simulink model "PendulumProjectMU"  (R2022b)
settings: Solver=FixedStepAuto  StartTime=0.0  StopTime=inf  FixedStep=0.01  RelTol=1e-3
model workspace (MATLAB code in the model file):
  | %Parameters from hardware:
  | Mc = 0.540 + 0.048;% [kg]mass of cart
  | l = 0.49; % [m] Pendelum length
  | Lcg = l/2; % [m] lenght to center of mass
  | m = 0.022;% [kg] Mass of pendelum rod
  | g = 9.81; % m/s^2
  | 
  | %Motor parameters (some estimates, some from Sonali):
  | Rm = 1.3;%[ohm] motor armature resistence
  | kb = 0.02;%[vs/rad]back emf constant
  | kt = 0.02;%[vs/rad]motor touque constant
  | r =  0.04/(2*pi); %[m]radius pulley motor (and encoder)
  | 
  | %Very rough estimate:
  | c = 5; %[N/(m/s)] viscous friction cart
  | b = 0.00001;% [Nm/rad/s]Viscous damping pendelum
  | I = 0.00007; % [kgm^2]
  | 
  | %FOR CASE LOGIC SIMULINK MODEL:
  | offset= 15;% degrees Ofsett from pi, before pendelum control takes over for swing up
  | highThetaTreshold = pi+ pi*offset/180;
  | lowThetaTreshold = pi- pi*offset/180;
  | 
  | %Theshold values to stop cart if close to edges
  | xMAX = 0.25;
  | xMIN = -0.25;
libraries: arduinolib x8, simulink x2, arduinosensorlib x2
settings Model: FPTRunName=Active  ExtModeTrigDuration=2  Creator=The MathWorks, Inc.  LastModifiedBy=Bruker
settings SolverCC: AlgebraicLoopSolver=TrustRegion
settings DataIOCC: LimitDataPoints=on  ReturnWorkspaceOutputs=off
settings OptimizationCC: ExpressionDepthLimit=2147483647  LifeSpan=Inf  MaxStackSize=64
settings DebuggingCC: UnderspecifiedInitializationDetection=Classic  MergeDetectMultiDrivingBlocksExec=none  FcnCallInpInsideContextMsg=warning  UnconnectedInputMsg=warning  UnconnectedOutputMsg=warning  UnconnectedLineMsg=warning  AllowSymbolicDim=off  StateNameClashWarn=warning  SFUnexpectedBacktrackingDiag=warning  SFNoUnconditionalDefaultTransitionDiag=warning  SFExecutionAtInitializationDiag=none  SFMachineParentedDataDiag=warning  ArithmeticOperatorsInVariantConditions=warning
settings HardwareCC: ProdBitPerInt=16  ProdBitPerPointer=16  ProdBitPerSizeT=16  ProdBitPerPtrDiffT=16  ProdLargestAtomicFloat=None  ProdWordSize=8  ProdHWDeviceType=Atmel->AVR  UseEmbeddedCoderFeatures=off  UseSimulinkCoderFeatures=off
settings ModelReferenceCC: EnableRefExpFcnMdlSchedulingChecks=on
settings SFSimCC: SimUseLocalCustomCode=off  MATLABDynamicMemAlloc=off
settings RTWCC: Description=Embedded Coder  SystemTargetFile=ert.tlc  HardwareBoard=Arduino Mega 2560  TemplateMakefile=ert_default_tmf  GenerateReport=on  RTWVerbose=off  RTWUseLocalCustomCode=off  Toolchain=Arduino AVR  BuildConfiguration=Faster Runs  LaunchReport=on  DLArmComputeVersion=19.05
settings CodeAppCC: ForceParamTrailComments=on  OperatorAnnotations=on  MangleLength=10  StateflowObjectComments=on  MATLABSourceComments=on
settings ERTTargetCC: MultiwordLength=2048  ERTCustomFileBanners=off  SupportContinuousTime=on  SupportNonInlinedSFcns=on  RemoveResetFunc=off  ModelStepFunctionPrototypeControlCompliant=off
settings ConfigComp: CovMetricSettings=dw  CovSaveCumulativeToWorkspaceVar=on  CovSaveSingleToWorkspaceVar=on  CovExternalEMLEnable=off  CovSFcnEnable=off

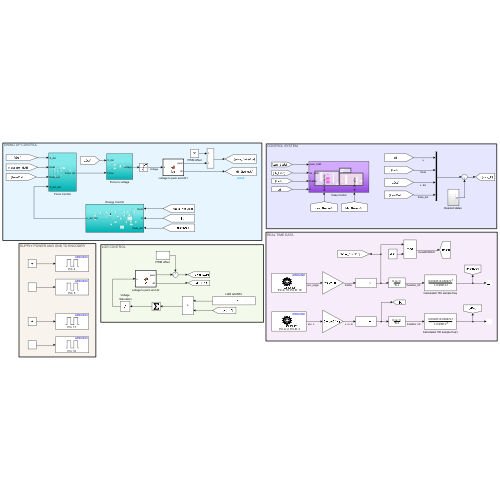
[thumbnail: Simulink's stored preview of the top-level diagram]
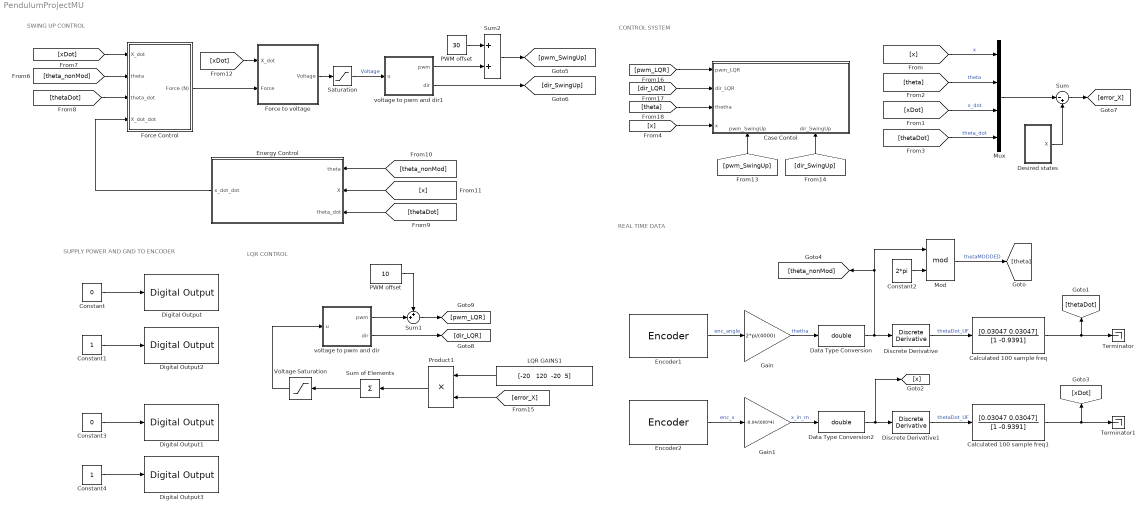
== system PendulumProjectMU ==
  note: LQR CONTROL
  note: SWING UP CONTROL
  note: CONTROL SYSTEM
  note: REAL TIME DATA
  note: SUPPLY POWER AND GND TO ENCODER
  Calculated 100 sample freq : DiscreteFilter  Numerator=[0.03047 0.03047]  Denominator=[1 -0.9391]  SampleTime=0.01
  Calculated 100 sample freq1 : DiscreteFilter  Numerator=[0.03047 0.03047]  Denominator=[1 -0.9391]  SampleTime=0.01
  Case Contol : Subsystem
      settings: PortSchema="{\"entries\":[{\"content\":{\"sides\":[{\"content\":{\"connectorIds\":[\"In1\",\"In2\",\"In3\",\"In4\"]},\"type\":\"ConnectorPlacement.EquallySpacedRectSide\",\"uuid\":\"b9c187f4-b904-4d2f-9cde-60dd328b1521\"},{\"content\":{\"connectorIds\":[],\"side\":\"RIGHT\"},\"type\":\"ConnectorPlacement.EquallySpacedRectSide\",\"uuid\":\"bc2320ec-c90b-418d-8662-363a4a51a6b8\"},{\"content\":{\"connectorIds\":[],\"side\":\"TOP\"},\"type\":\"ConnectorPlacement.EquallySpacedRectSide\",\"uuid\":\"d413f3a0-4126-4ff6-b863-89d2afe3c2f6\"},{\"content\":{\"connectorIds\":[\"In5\",\"In6\"],\"side\":\"BOTTOM\"},\"type\":\"ConnectorPlacement.EquallySpacedRectSide\",\"uuid\":\"5bcc0f4c-eb85-4f39-a4e6-dc5e871715b7\"}]},\"type\":\"ConnectorPlacement.EquallySpacedConnector\",\"uuid\":\"881b5d2a-3ec5-43c5-91bc-30ecaf4ea49e\"}],\"packageUris\":[\"http://schema.mathworks.com/mf0/Connector/R2020b\"],\"version\":\"1.0\"}"
  Constant : Constant  Value=0
  Constant1 : Constant
  Constant2 : Constant  Value=2*pi
  Constant3 : Constant  Value=0
  Constant4 : Constant
  Data Type Conversion : DataTypeConversion  OutDataTypeStr=double  SaturateOnIntegerOverflow=off  RndMeth=Floor
  Data Type Conversion2 : DataTypeConversion  OutDataTypeStr=double  SaturateOnIntegerOverflow=off  RndMeth=Floor
  "Desired states " : Subsystem
  Digital Output : arduinolib/Digital Output  pinNumber=4  Direction=output  blockPlatform=arduino
  Digital Output1 : arduinolib/Digital Output  pinNumber=17  Direction=output  blockPlatform=arduino
  Digital Output2 : arduinolib/Digital Output  pinNumber=5  Direction=output  blockPlatform=arduino
  Digital Output3 : arduinolib/Digital Output  pinNumber=16  Direction=output  blockPlatform=arduino
  Discrete Derivative : simulink/Quick Insert/Discrete/Discrete Derivative  gainval=1.0  ICPrevScaledInput=0.0  OutMin=[]  OutMax=[]  OutDataType=fixdt(1, 16)  OutScaling=2^-10  DoSatur=off
  Discrete Derivative1 : simulink/Quick Insert/Discrete/Discrete Derivative  gainval=1.0  ICPrevScaledInput=0.0  OutMin=[]  OutMax=[]  OutDataType=fixdt(1, 16)  OutScaling=2^-10  DoSatur=off
  Encoder1 : arduinosensorlib/Encoder  InputA=19  InputB=18  Mode=No reset  SampleTime=0.01
  Encoder2 : arduinosensorlib/Encoder  InputA=2  InputB=3  Mode=No reset  SampleTime=0.01
  Energy Control : Subsystem
  Force Control : Subsystem
  Force to voltage : Subsystem
  Gain : Gain  Gain=2*pi/(4000)
  Gain1 : Gain  Gain=-0.04/(600*4)
  LQR GAINS1 : Constant  Value="[-20   120  -20  5]"
  Mod : Math  Operator=mod  SignedPower=on
  Mux : Mux
  PWM offset : Constant  Value=30
  "PWM offset " : Constant  Value=10
  Product1 : Product
  Saturation : Saturate  UpperLimit=3.2  LowerLimit=-3.2
  Sum : Sum  Inputs=|-+
  Sum of Elements : Sum  Inputs=+
  Sum1 : Sum  Inputs=++|
  Sum2 : Sum
  Terminator : Terminator
  Terminator1 : Terminator
  Voltage Saturation : Saturate  UpperLimit=6  LowerLimit=-6
  voltage to pwm and dir : MATLAB Function  TreatAsAtomicUnit=on
  voltage to pwm and dir1 : MATLAB Function  TreatAsAtomicUnit=on
  wires:
  Encoder1/1 -> Gain/1  "enc_angle"
  Constant/1 -> Digital Output/1
  Constant1/1 -> Digital Output2/1
  Gain/1 -> Data Type Conversion/1  "thetha"
  Encoder2/1 -> Gain1/1  "enc_x"
  Constant3/1 -> Digital Output1/1
  Constant4/1 -> Digital Output3/1
  Gain1/1 -> Data Type Conversion2/1  "x_in_m"
  [theta] -> Mux/2  "theta"
  [x] -> Mux/1  "x"
  Mux/1 -> Sum/1
  [xDot] -> Mux/3  "x_dot"
  [thetaDot] -> Mux/4  "theta_dot"
  Data Type Conversion2/1 -> Discrete Derivative1/1, [x]
  Voltage Saturation/1 -> voltage to pwm and dir/1(u)
  voltage to pwm and dir/1(pwm) -> Sum1/2
  "PWM offset "/1 -> Sum1/1
  Calculated 100 sample freq1/1 -> [xDot], Terminator1/1
  Calculated 100 sample freq/1 -> [thetaDot], Terminator/1
  Discrete Derivative/1 -> Calculated 100 sample freq/1  "thetaDot_UF"
  Discrete Derivative1/1 -> Calculated 100 sample freq1/1  "thetaDot_UF"
  "Desired states "/1(X) -> Sum/2
  [theta] -> Case Contol/3(thetha)
  Data Type Conversion/1 -> Discrete Derivative/1, Mod/1, [theta_nonMod]
  Mod/1 -> [theta]  "thetaMODDED"
  [x] -> Case Contol/4(x)
  Force to voltage/1(Voltage) -> Saturation/1
  Energy Control/1(x_dot_dot) -> Force Control/4(X_dot_dot)
  Force Control/1(Force (N)) -> Force to voltage/2(Force)
  [theta_nonMod] -> Force Control/2(theta)
  [xDot] -> Force Control/1(X_dot)
  [thetaDot] -> Force Control/3(theta_dot)
  [thetaDot] -> Energy Control/3(theta_dot)
  [theta_nonMod] -> Energy Control/1(theta)
  [x] -> Energy Control/2(X)
  [xDot] -> Force to voltage/1(X_dot)
  Saturation/1 -> voltage to pwm and dir1/1(u)  "Voltage"
  Product1/1 -> Sum of Elements/1
  LQR GAINS1/1 -> Product1/1
  Sum of Elements/1 -> Voltage Saturation/1
  PWM offset/1 -> Sum2/1
  voltage to pwm and dir1/1(pwm) -> Sum2/2
  Sum2/1 -> [pwm_SwingUp]
  voltage to pwm and dir1/2(dir) -> [dir_SwingUp]
  [pwm_SwingUp] -> Case Contol/5(pwm_SwingUp)
  [dir_SwingUp] -> Case Contol/6(dir_SwingUp)
  Sum/1 -> [error_X]
  [error_X] -> Product1/2
  voltage to pwm and dir/2(dir) -> [dir_LQR]
  Sum1/1 -> [pwm_LQR]
  [pwm_LQR] -> Case Contol/1(pwm_LQR)
  [dir_LQR] -> Case Contol/2("dir_LQR ")
  Constant2/1 -> Mod/2

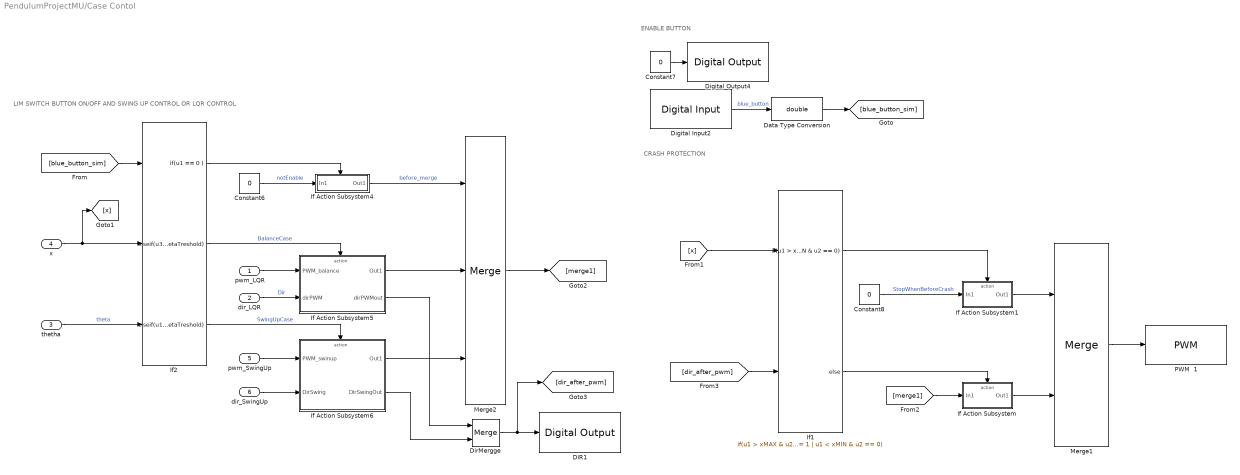
== system PendulumProjectMU/Case Contol ==
  note: CRASH PROTECTION
  note: ENABLE BUTTON
  note: LIM SWITCH BUTTON ON/OFF AND SWING UP CONTROL OR LQR CONTROL
  pwm_LQR : Inport
  "dir_LQR " : Inport  Port=2
  thetha : Inport  Port=3
  x : Inport  Port=4
  pwm_SwingUp : Inport  Port=5
  dir_SwingUp : Inport  Port=6
  Constant6 : Constant  Value=0
  Constant7 : Constant  Value=0
  Constant8 : Constant  Value=0
  DIR1 : arduinolib/Digital Output  pinNumber=12  Direction=output  blockPlatform=arduino
  Data Type Conversion : DataTypeConversion  OutDataTypeStr=double  SaturateOnIntegerOverflow=off  RndMeth=Floor
  Digital Input2 : arduinolib/Digital Input  pinNumber=42  mode=Input Pullup  Direction=input  SampleTime=0.01  blockPlatform=arduino
  Digital Output4 : arduinolib/Digital Output  pinNumber=43  Direction=output  blockPlatform=arduino
  DirMergge : Merge
  If Action Subsystem : Subsystem  TreatAsAtomicUnit=on
  If Action Subsystem1 : Subsystem  TreatAsAtomicUnit=on
  If Action Subsystem4 : Subsystem  TreatAsAtomicUnit=on
  If Action Subsystem5 : Subsystem  TreatAsAtomicUnit=on
  If Action Subsystem6 : Subsystem  TreatAsAtomicUnit=on
  If1 : If  NumInputs=2  IfExpression=u1 > xMAX & u2 == 1 | u1 < xMIN & u2 == 0
  If2 : If  NumInputs=3  IfExpression=u1 == 0  ElseIfExpressions="u3 < highThetaTreshold & u3 > lowThetaTreshold  , u1 ~= 0  & u3 > highThetaTreshold | u3 < lowThetaTreshold"  ShowElse=off
  Merge1 : Merge
  Merge2 : Merge  Inputs=3
  PWM  1 : arduinolib/PWM  pinNumber=13  frequencyType=Default  desiredFrequency=490.2  achievableFrequency=490.2
  wires:
  Constant7/1 -> Digital Output4/1
  If2/3 -> If Action Subsystem6/Action  "SwingUpCase"
  If Action Subsystem4/1(Out1) -> Merge2/1  "before_merge"
  If2/1 -> If Action Subsystem4/Action
  Constant6/1 -> If Action Subsystem4/1(In1)  "notEnable"
  Digital Input2/1 -> Data Type Conversion/1  "blue_button"
  If Action Subsystem6/1(Out1) -> Merge2/3
  If Action Subsystem5/1(Out1) -> Merge2/2
  thetha/1 -> If2/3  "theta"
  pwm_LQR/1 -> If Action Subsystem5/1(PWM_balance)
  x/1 -> [x], If2/2
  pwm_SwingUp/1 -> If Action Subsystem6/1(PWM_swinup)
  "dir_LQR "/1 -> If Action Subsystem5/2(dirPWM)  "Dir"
  dir_SwingUp/1 -> If Action Subsystem6/2(DirSwing)
  If Action Subsystem5/2(dirPWMout) -> DirMergge/1
  If Action Subsystem6/2(DirSwingOut) -> DirMergge/2
  If1/1 -> If Action Subsystem1/Action
  Constant8/1 -> If Action Subsystem1/1(In1)  "StopWhenBeforeCrash"
  If1/2 -> If Action Subsystem/Action
  If Action Subsystem1/1(Out1) -> Merge1/1
  If Action Subsystem/1(Out1) -> Merge1/2
  Merge1/1 -> PWM  1/1
  If2/2 -> If Action Subsystem5/Action  "BalanceCase"
  Data Type Conversion/1 -> [blue_button_sim]
  [blue_button_sim] -> If2/1
  [x] -> If1/1
  Merge2/1 -> [merge1]
  [merge1] -> If Action Subsystem/1(In1)
  [dir_after_pwm] -> If1/2
  DirMergge/1 -> [dir_after_pwm], DIR1/1

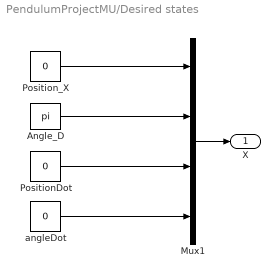
== system PendulumProjectMU/Desired states  ==
  Angle_D : Constant  Value=pi
  Mux1 : Mux
  PositionDot : Constant  Value=0
  Position_X : Constant  Value=0
  angleDot : Constant  Value=0
  X : Outport  VectorParamsAs1DForOutWhenUnconnected=off
  wires:
  Position_X/1 -> Mux1/1
  Angle_D/1 -> Mux1/2
  angleDot/1 -> Mux1/4
  PositionDot/1 -> Mux1/3
  Mux1/1 -> X/1

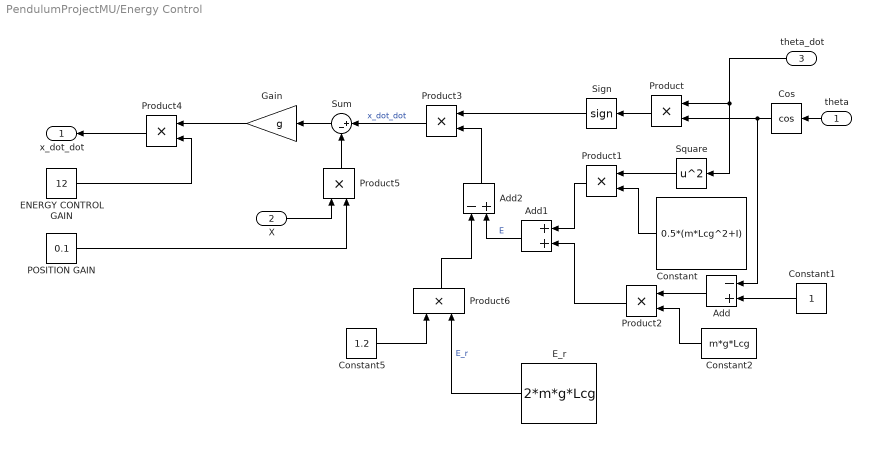
== system PendulumProjectMU/Energy Control ==
  theta : Inport
  X : Inport  Port=2
  theta_dot : Inport  Port=3
  Add : Sum  Inputs=-+
  Add1 : Sum
  Add2 : Sum  Inputs=-+
  Constant : Constant  Value=0.5*(m*Lcg^2+I)  SampleTime=0.01
  Constant1 : Constant  SampleTime=0.01
  Constant2 : Constant  Value=m*g*Lcg
  Constant5 : Constant  Value=1.2  SampleTime=0.01
  Cos : Trigonometry  Operator=cos
  ENERGY CONTROL GAIN : Constant  Value=12  SampleTime=0.01
  E_r : Constant  Value=2*m*g*Lcg  SampleTime=0.01
  Gain : Gain  Gain=g
  POSITION GAIN : Constant  Value=0.1  SampleTime=0.01
  Product{,1..6} (7 alike) : Product
  Sign : Signum
  Square : Math  Operator=square
  Sum : Sum  Inputs=|+-
  x_dot_dot : Outport
  wires:
  E_r/1 -> Product6/2  "E_r"
  Constant/1 -> Product1/2
  Sign/1 -> Product3/1
  Constant2/1 -> Product2/2
  theta_dot/1 -> Square/1, Product/1
  Add/1 -> Product2/1
  Product/1 -> Sign/1
  Add1/1 -> Add2/2  "E"
  Cos/1 -> Product/2, Add/1
  Square/1 -> Product1/1
  Constant1/1 -> Add/2
  Product2/1 -> Add1/2
  Product1/1 -> Add1/1
  Add2/1 -> Product3/2
  theta/1 -> Cos/1
  Product4/1 -> x_dot_dot/1
  Sum/1 -> Gain/1
  Product3/1 -> Sum/1  "x_dot_dot"
  X/1 -> Product5/1
  Product6/1 -> Add2/1
  Product5/1 -> Sum/2
  POSITION GAIN/1 -> Product5/2
  Constant5/1 -> Product6/1
  Gain/1 -> Product4/1
  ENERGY CONTROL GAIN/1 -> Product4/2

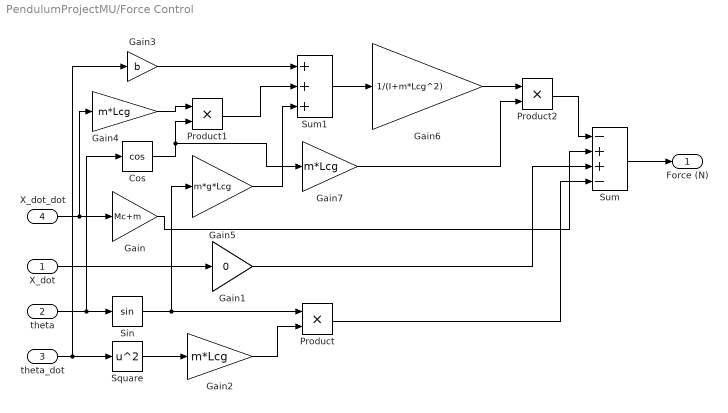
== system PendulumProjectMU/Force Control ==
  X_dot : Inport
  theta : Inport  Port=2
  theta_dot : Inport  Port=3
  X_dot_dot : Inport  Port=4
  Cos : Trigonometry  Operator=cos
  Gain : Gain  Gain=Mc+m
  Gain1 : Gain  Gain=0
  Gain2 : Gain  Gain=m*Lcg
  Gain3 : Gain  Gain=b
  Gain4 : Gain  Gain=m*Lcg
  Gain5 : Gain  Gain=m*g*Lcg
  Gain6 : Gain  Gain=1/(I+m*Lcg^2)
  Gain7 : Gain  Gain=m*Lcg
  Product : Product
  Product1 : Product
  Product2 : Product
  Sin : Trigonometry
  Square : Math  Operator=square
  Sum : Sum  Inputs=-++-
  Sum1 : Sum  Inputs=+++
  Force (N) : Outport  VectorParamsAs1DForOutWhenUnconnected=off
  wires:
  X_dot_dot/1 -> Gain/1, Gain4/1
  X_dot/1 -> Gain1/1
  Square/1 -> Gain2/1
  theta/1 -> Cos/1, Sin/1
  Sin/1 -> Gain5/1, Product/1
  Gain2/1 -> Product/2
  Product/1 -> Sum/4
  Gain1/1 -> Sum/3
  Gain/1 -> Sum/2
  Gain3/1 -> Sum1/1
  Gain4/1 -> Product1/1
  Cos/1 -> Gain7/1, Product1/2
  theta_dot/1 -> Square/1, Gain3/1
  Product1/1 -> Sum1/2
  Gain5/1 -> Sum1/3
  Sum1/1 -> Gain6/1
  Gain6/1 -> Product2/1
  Gain7/1 -> Product2/2
  Product2/1 -> Sum/1
  Sum/1 -> Force (N)/1

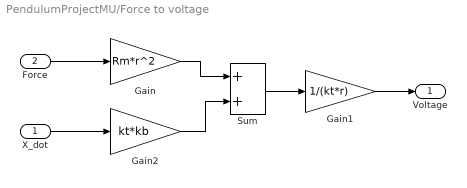
== system PendulumProjectMU/Force to voltage ==
  X_dot : Inport
  Force : Inport  Port=2
  Gain : Gain  Gain=Rm*r^2
  Gain1 : Gain  Gain=1/(kt*r)
  Gain2 : Gain  Gain=kt*kb
  Sum : Sum
  Voltage : Outport
  wires:
  X_dot/1 -> Gain2/1
  Force/1 -> Gain/1
  Gain/1 -> Sum/1
  Gain2/1 -> Sum/2
  Sum/1 -> Gain1/1
  Gain1/1 -> Voltage/1

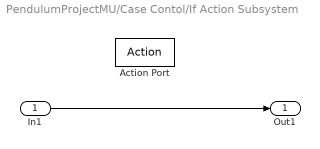
== system PendulumProjectMU/Case Contol/If Action Subsystem ==
  In1 : Inport
  Action Port : ActionPort  ActionPortLabel=else
  Out1 : Outport
  wires:
  In1/1 -> Out1/1

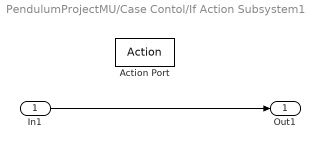
== system PendulumProjectMU/Case Contol/If Action Subsystem1 ==
  In1 : Inport
  Action Port : ActionPort  ActionPortLabel=if(u1 > xMAX & u2 == 1 | u1 < xMIN & u2 == 0)
  Out1 : Outport
  wires:
  In1/1 -> Out1/1

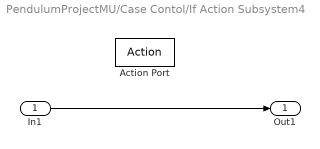
== system PendulumProjectMU/Case Contol/If Action Subsystem4 ==
  In1 : Inport
  Action Port : ActionPort  ActionPortLabel=if(u1 == 0 )
  Out1 : Outport
  wires:
  In1/1 -> Out1/1

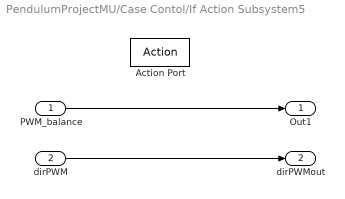
== system PendulumProjectMU/Case Contol/If Action Subsystem5 ==
  PWM_balance : Inport
  dirPWM : Inport  Port=2
  Action Port : ActionPort  ActionPortLabel="elseif(u3 < highThetaTreshold & u3 > lowThetaTreshold  )"
  Out1 : Outport
  dirPWMout : Outport  Port=2
  wires:
  PWM_balance/1 -> Out1/1
  dirPWM/1 -> dirPWMout/1

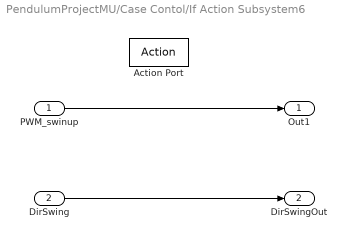
== system PendulumProjectMU/Case Contol/If Action Subsystem6 ==
  PWM_swinup : Inport
  DirSwing : Inport  Port=2
  Action Port : ActionPort  ActionPortLabel="elseif( u1 ~= 0  & u3 > highThetaTreshold | u3 < lowThetaTreshold)"
  Out1 : Outport
  DirSwingOut : Outport  Port=2
  wires:
  PWM_swinup/1 -> Out1/1
  DirSwing/1 -> DirSwingOut/1

== matlab function PendulumProjectMU/voltage to pwm and dir1 ==
  data: pwm output; u input; dir output
function [pwm, dir]  = fcn(u)

signx = sign(u);
pwm = abs(u)/12*255; %Converts from voltage to PWM

if(signx<0)
    dir = 0;
else
    dir = 1;
end

end

== matlab function PendulumProjectMU/voltage to pwm and dir ==
  data: pwm output; u input; dir output
function [pwm, dir]  = fcn(u)

signx = sign(u);
pwm = abs(u)/12*255; %Converts from voltage to PWM

if(signx<0)
    dir = 0;
else
    dir = 1;
end

end
